simulink model "RS_Code"  (R2018a)
settings: Solver=VariableStepAuto  StartTime=0.0  StopTime=100000  RelTol=1e-3
values from neighbouring files (symbols this model uses):
  RS_EbNoUncoded = 13    [RS_code_simulimk.m]
  RS_k = 53    [RS_code_simulimk.m]
  RS_n = 63    [RS_code_simulimk.m]
  RS_numBitsPerSymbol = log2(RS_MQAM)    [RS_code_simulimk.m]
  RS_TsUncoded = 1    [RS_code_simulimk.m]
undefined symbols (not defined in the file or in its folder): rsgenpoly
libraries: commblkcod2 x2, commdigbbndam3 x2, commchan3 x1, dspmathops x1, commsink2 x1, commrandsrc3 x1
settings Model: Creator=Hassan  LastModifiedBy=Hassan

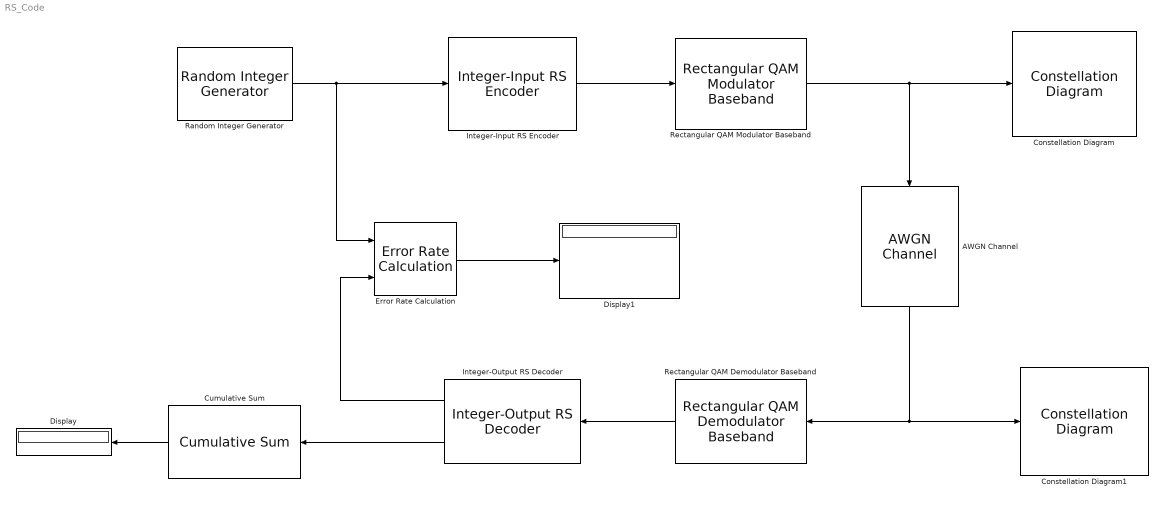
== system RS_Code ==
  AWGN Channel : commchan3/AWGN Channel  InputProcessing=Columns as channels (frame based)  seed=67  noiseMode="Signal to noise ratio  (Eb/No)"  EbNodB=RS_EbNoUncoded + 10*log10(RS_k/RS_n)  EsNodB=10  SNRdB=RS_EbNoUncoded+10*log(RS_k/RS_n)+10*log(RS_numBitsPerSymbol)  bitsPerSym=RS_numBitsPerSymbol  Ps=RS_sigPower  Tsym=RS_TsUncoded * (RS_k/RS_n)  variance=1
  Constellation Diagram : ConstellationDiagram
  Constellation Diagram1 : ConstellationDiagram
  Cumulative Sum : dspmathops/Cumulative Sum  dim=Channels (running sum)  InputProcessing=Columns as channels (frame based)  reset_popup=None  roundingMode=Floor  overflowMode=off  outputDataTypeStr=Inherit: Same as accumulator  outputMin=[]  outputMax=[]  outputLastDataTypeStr=Inherit: Same as accumulator
      settings: SourceProductName=DSP System Toolbox
  Display : Display
  Display1 : Display
  Error Rate Calculation : commsink2/Error Rate Calculation  N=0  st_delay=0  cp_mode=Entire frame  subframe=[]  PMode=Port  WsName=ErrorVec  RsMode2=off  stop=off  numErr=100  maxBits=1e6
  Integer-Input RS Encoder : commblkcod2/Integer-Input RS Encoder  n=RS_n  k=RS_k  specShortening=off  shortenedK=3  specGenPoly=off  genPoly=rsgenpoly(7, 3, [], [], 'double')  specPrimPoly=off  prPoly='X^3 + X + 1'  specPuncture=off  punctVec=[ones(2,1); zeros(2,1)]
      settings: SourceProductName=Communications System Toolbox  SourceProductBaseCode=CM
  Integer-Output RS Decoder : commblkcod2/Integer-Output RS Decoder  n=RS_n  k=RS_k  specShortening=off  shortenedK=3  specGenPoly=off  genPoly=rsgenpoly(7, 3, [], [], 'double')  specPrimPoly=off  prPoly='X^3 + X + 1'  specPuncture=off  punctVec=[ones(2,1); zeros(2,1)]  specErasurePort=off  showNumErr=on
      settings: SourceProductName=Communications System Toolbox  SourceProductBaseCode=CM
  Random Integer Generator : commrandsrc3/Random Integer Generator  SetSize=RS_MQAM  SeedSource=Parameter  Seed=37  SampleTime=RS_TsUncoded  SamplesPerFrame=RS_k  OutputDataType=double  SimulateUsing=Interpreted execution
  Rectangular QAM Demodulator Baseband : commdigbbndam3/Rectangular QAM Demodulator Baseband  M=RS_MQAM  OutType=Integer  DecType=Hard decision  VarSource=Dialog  Variance=1  Dec=Gray  Mapping=[0:15]  PowType=Average Power  MinDist=2  AvgPow=RS_sigPower  PeakPow=1  Ph=0  outDtype1=Inherit via internal rule  outDtype2=Inherit via internal rule  derotateFactorWordLen=16  derotateFactorDataTypeStr=Inherit: Same word length as input  derotateFactorLastDataTypeStr=Inherit: Same word length as input  denormFactorWordLen=16  denormFactorDataTypeStr=Inherit: Same word length as input  denormFactorLastDataTypeStr=Inherit: Same word length as input  prodOutWordLen=32  prodOutOverflowMode=Wrap  prodOutRoundingMode=Floor  prodOutOvFlMode=off  prodOutOvFlModeLastStrValue=off  sumWordLen=32
  Rectangular QAM Modulator Baseband : commdigbbndam3/Rectangular QAM Modulator Baseband  M=RS_MQAM  InType=Integer  Enc=Gray  Mapping=[0:15]  PowType=Average Power  MinDist=2  AvgPow=RS_sigPower  PeakPow=1  Ph=0  outDtype=double  outWordLen=16  outUDDataType=sfix(16)  outFracLenMode=Best precision  outFracLen=15  outDataTypeStr=double  outLastDataTypeStr=double
  wires:
  Random Integer Generator/1 -> Error Rate Calculation/1, Integer-Input RS Encoder/1
  Integer-Input RS Encoder/1 -> Rectangular QAM Modulator Baseband/1
  Rectangular QAM Modulator Baseband/1 -> AWGN Channel/1, Constellation Diagram/1
  AWGN Channel/1 -> Rectangular QAM Demodulator Baseband/1, Constellation Diagram1/1
  Rectangular QAM Demodulator Baseband/1 -> Integer-Output RS Decoder/1
  Integer-Output RS Decoder/2 -> Cumulative Sum/1
  Cumulative Sum/1 -> Display/1
  Error Rate Calculation/1 -> Display1/1
  Integer-Output RS Decoder/1 -> Error Rate Calculation/2
